simulink subsystem "Gyrostellar_KF"  (R2021a)
settings: Solver=VariableStepAuto  StartTime=0.0  StopTime=10.0  RelTol=1e-3
undefined symbols (not defined in the file): gyro_bias_init, init_align_error, magnitude
libraries: dspmtrx3 x1
settings Model: Creator=Laura  LastModifiedBy=Laura

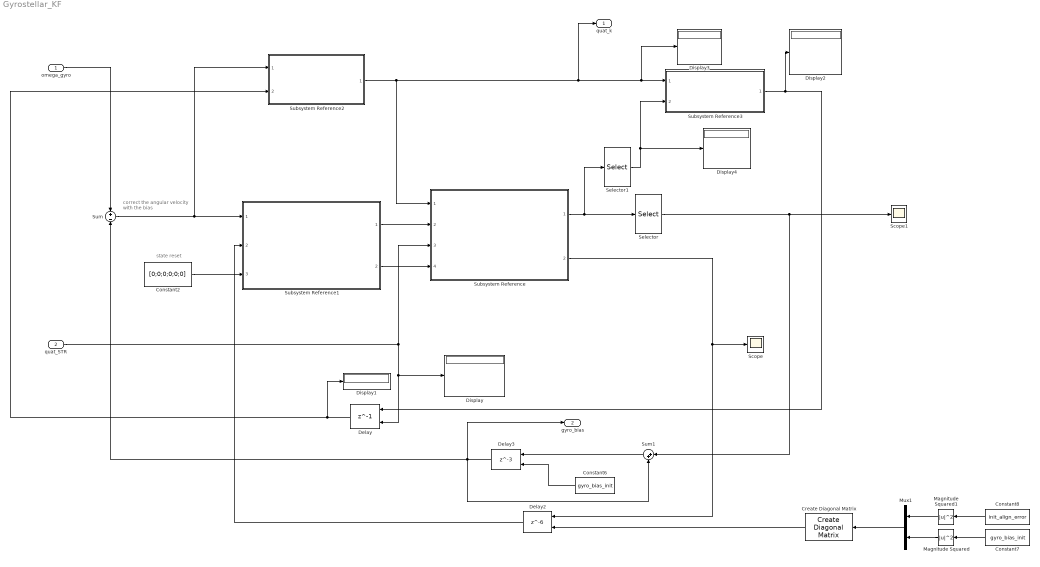
== system Gyrostellar_KF ==
  note: correct the angular velocity with the bias
  note: state reset
  omega_gyro : Inport  SampleTime=1/40
  quat_STR : Inport  Port=2  SampleTime=1/40
  Constant2 : Constant  Value=[0;0;0;0;0;0]
  Constant6 : Constant  Value=gyro_bias_init
  Constant7 : Constant  Value=gyro_bias_init
  Constant8 : Constant  Value=init_align_error
  Create Diagonal Matrix : dspmtrx3/Create Diagonal Matrix
      settings: SourceProductBaseCode=DS
  Delay : Delay  DelayLength=1  InitialConditionSource=Input port  SampleTime=1/10
      settings: InputPortMap=u0,p4
  Delay2 : Delay  DelayLength=6  InitialConditionSource=Input port  InputProcessing=Columns as channels (frame based)  SampleTime=1/40
      settings: InputPortMap=u0,p4
  Delay3 : Delay  DelayLength=3  InitialConditionSource=Input port  InputProcessing=Columns as channels (frame based)  SampleTime=1/10
      settings: InputPortMap=u0,p4
  Display{,1..4} (5 alike) : Display
  Magnitude Squared : Math  Operator=magnitude^2  SaturateOnIntegerOverflow=on
  Magnitude Squared1 : Math  Operator=magnitude^2  SaturateOnIntegerOverflow=on
  Mux1 : Mux  Inputs=2
  Scope : Scope
  Scope1 : Scope
  Selector : Selector  InputPortWidth=6  IndexOptions=Index vector (dialog)  Indices=[4 5 6]  OutputSizes=1
  Selector1 : Selector  InputPortWidth=6  IndexOptions=Index vector (dialog)  Indices=[1 2 3]  OutputSizes=1
  Subsystem Reference : Subsystem  ReferencedSubsystem=KF_update
  Subsystem Reference1 : Subsystem  ReferencedSubsystem=KF_prediction
  Subsystem Reference2 : Subsystem  ReferencedSubsystem=GyroIntegrator
  Subsystem Reference3 : Subsystem  ReferencedSubsystem=QuaternionUpdate
  Sum : Sum  Inputs=+-
  Sum1 : Sum  Inputs=|++
  quat_k : Outport  SampleTime=1/40  LockScale=on
  gyro_bias : Outport  Port=2
  wires:
  omega_gyro/1 -> Sum/1
  Subsystem Reference1/1 -> Subsystem Reference/2
  Subsystem Reference1/2 -> Subsystem Reference/4
  Constant2/1 -> Subsystem Reference1/3
  Subsystem Reference/1 -> Selector1/1, Selector/1
  Selector1/1 -> Display4/1, Subsystem Reference3/2
  Subsystem Reference3/1 -> Delay/1, Display2/1
  Sum/1 -> Subsystem Reference1/1, Subsystem Reference2/1
  Delay2/1 -> Subsystem Reference1/2
  quat_STR/1 -> Subsystem Reference/3, Display/1, Delay/2
  Constant7/1 -> Magnitude Squared/1
  Create Diagonal Matrix/1 -> Delay2/2
  Magnitude Squared/1 -> Mux1/2
  Magnitude Squared1/1 -> Mux1/1
  Constant8/1 -> Magnitude Squared1/1
  Mux1/1 -> Create Diagonal Matrix/1
  Subsystem Reference2/1 -> Subsystem Reference3/1, Display3/1, quat_k/1, Subsystem Reference/1
  Subsystem Reference/2 -> Delay2/1, Scope/1
  Selector/1 -> Sum1/1, Scope1/1
  Sum1/1 -> Delay3/1
  Constant6/1 -> Delay3/2
  Delay/1 -> Subsystem Reference2/2, Display1/1
  Delay3/1 -> Sum/2, gyro_bias/1, Sum1/2
